simulink model "trafficLight"  (R2025b)
settings: Solver=FixedStepDiscrete  StartTime=0.0  StopTime=500  FixedStep=1  RelTol=1e-3
settings Model: DataTypeOverride=Off  PacingRate=28  Creator=Soochan Kim  LastModifiedBy=Soochan Kim
settings OptimizationCC: BlockReduction=off  ConditionallyExecuteInputs=off  DefaultParameterBehavior=Inlined  InheritOutputTypeSmallerThanSingle=on
settings DebuggingCC: ArtificialAlgebraicLoopMsg=error  SingleTaskRateTransMsg=error
settings HardwareCC: ProdBitPerPointer=32.0  ProdBitPerSizeT=32.0  ProdBitPerPtrDiffT=32.0  ProdLargestAtomicFloat=None  ProdIntDivRoundTo=Undefined  ProdEndianess=Unspecified  ProdWordSize=32.0  ProdHWDeviceType=ASIC/FPGA->ASIC/FPGA  TargetBitPerPointer=64.0  TargetBitPerSizeT=64.0  TargetBitPerPtrDiffT=64.0  TargetLongLongMode=on  TargetIntDivRoundTo=Zero  TargetEndianess=LittleEndian  TargetWordSize=64.0  TargetHWDeviceType=Custom Processor->MATLAB Host Computer  ProdEqTarget=off

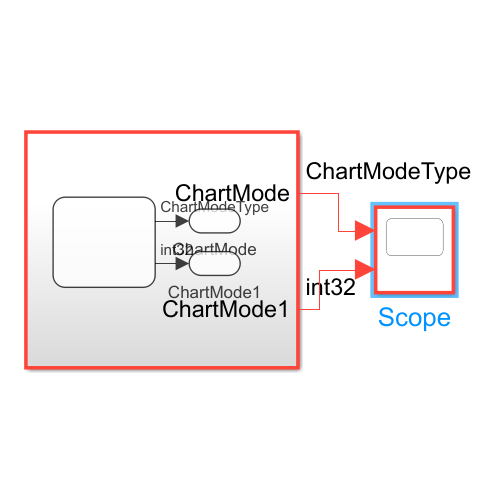
[thumbnail: Simulink's stored preview of the top-level diagram]
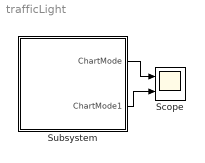
== system trafficLight ==
  Scope : Scope  NumInputPorts=2
      settings: ActiveDisplayYMinimum=0.75000000000000011  ActiveDisplayYMaximum=3.25
  Subsystem : Subsystem
  wires:
  Subsystem/1(ChartMode) -> Scope/1
  Subsystem/2(ChartMode1) -> Scope/2

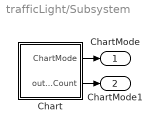
== system trafficLight/Subsystem ==
  Chart : Stateflow chart  TreatAsAtomicUnit=on
  ChartMode : Outport
  ChartMode1 : Outport  Port=2
  wires:
  Chart/1(ChartMode) -> ChartMode/1
  Chart/2(outRedHitCount) -> ChartMode1/1

== stateflow chart trafficLight/Subsystem/Chart ==
  settings: stateMachineType=MOORE_MACHINE  executeAtInitialization=1
  state Red
    outRedHitCount =  redHitCount;
    redHitCount = redHitCount + int32(1);
  state Green
  state Yello
  (default) -> Red
  Red -> Green : [after(90, sec)]
  Yello -> Red : [after(15,sec)]
  Green -> Yello : [after(65, sec)]
  data: ChartMode output Enum: ChartModeType; redHitCount local int32 =int32(1); outRedHitCount output =int32(0)
